simulink model "AUV_Multi_MPC"  (R2023a)
settings: Solver=ode23t  StartTime=0.0  StopTime=300  MaxStep=0.01  RelTol=1e-3  EnableMultiTasking=on
PreLoadFcn:
  | AUV_VehicleParameters;
  | Vehicle.Body.markeropacity = 0;
InitFcn:
  | %% ========================= SAMPLE TIME =========================
  | Ts = 0.1;
  | %% ========================= MPC: SURGE X =========================
  | nx = 1; nu = 1; ny = 1;
  | 
  | A = 0.9; B = 0.1; C = 1; D = 0;
  | plant = ss(A, B, C, D, Ts);
  | mpc1 = mpc(plant, Ts);
  | 
  | % Cấu hình như bình thường
  | mpc1.PredictionHorizon = 10;
  | mpc1.ControlHorizon = 2;
  | 
  | mpc1.Weights.OV = 7.5; % đủ mạnh để bám
  | mpc1.Weights.MV = 0.08; % cho dùng lực nhiều hơn
  | mpc1.Weights.MVRate = 0.25; % vừa mượt vừa linh hoạt
  | mpc1.MV.Min = -40;
  | mpc1.MV.Max = 40;
  | mpc1.OV.Min = 0;
  | mpc1.OV.Max = 2;
  | 
  | % Ràng buộc về thay đổi lực
  | mpc1.MV.RateMin = -12.5;
  | mpc1.MV.RateMax = 12.5;
  | %% ========================= MPC OUTER LOOP FOR DEPTH (Z) =========================
  | % ===== Baseline outer MPC for depth =====
  | u0 = 1.2;
  | 
  | A = 1;
  | B = -Ts*u0;
  | C = 1;
  | D = 0;
  | 
  | plant_z = ss(A,B,C,D,Ts);
  | 
  | mpc_z = mpc(plant_z,Ts);
  | mpc_z.PredictionHorizon = 10;
  | mpc_z.ControlHorizon    = 2;
  | 
  | mpc_z.Weights.OV     = 12;
  | mpc_z.Weights.MV     = 0.01;
  | mpc_z.Weights.MVRate = 0.1;
  | 
  | theta_ref_max = deg2rad(18);
  | mpc_z.MV.Min = -theta_ref_max;
  | mpc_z.MV.Max =  theta_ref_max;
  | 
  | mpc_z.MV.RateMin = -deg2rad(4);
  | mpc_z.MV.RateMax =  deg2rad(4);
  | 
  | 
  | %% ========================= MPC OUTER LOOP FOR HEADING =========================
  | A = 1;
  | B = Ts;
  | C = 1;
  | D = 0;
  | 
  | plant_psi = ss(A,B,C,D,Ts);
  | mpc_psi = mpc(plant_psi,Ts);
  | 
  | mpc_psi.PredictionHorizon = 10;
  | mpc_psi.ControlHorizon    = 2;
  | 
  | mpc_psi.Weights.OV     = 10;
  | mpc_psi.Weights.MV     = 0.05;
  | mpc_psi.Weights.MVRate = 1;
  | 
  | psidot_ref_max = deg2rad(20);
  | mpc_psi.MV.Min = -psidot_ref_max;
  | mpc_psi.MV.Max =  psidot_ref_max;
  | 
  | mpc_psi.MV.RateMin = -deg2rad(10);
  | mpc_psi.MV.RateMax =  deg2rad(10);
StopFcn:
  | try
  |     S = out;
  | 
  |     % ===============================
  |     % CHỌN HỆ QUY CHIẾU
  |     % ===============================
  |     USE_UP = true;   % true = ENU (Up), false = NED (Down)
  | 
  |     % ===============================
  |     % AUV position (NED gốc)
  |     % ===============================
  |     P  = squeeze(S.auv_position.signals.values);   % [Xn Ye Zd]
  |     tP = S.auv_position.time(:);
  | 
  |     Xn = P(:,1);   % North
  |     Ye = P(:,2);   % East
  |     Zd = P(:,3);   % Down (+)
  | 
  |     % ===============================
  |     % Reference vector
  |     % ===============================
  |     R = squeeze(S.auv_reference.signals.values);  % [V D psi]
  |     t = S.auv_reference.time(:);
  | 
  |     V   = R(:,1);      % speed
  |     D   = R(:,2);      % depth (Down +)
  |     psi = R(:,3);      % heading (rad)
  | 
  |     % ===============================
  |     % Reconstruct reference trajectory (NED)
  |     % ===============================
  |     Xr = Xn(1) + cumtrapz(t, V .* cos(psi));   % North
  |     Yr = Ye(1) + cumtrapz(t, V .* sin(psi));   % East
  |     Zr_down = Zd(1) + (D - D(1));              % Down (+)
  | 
  |     % ===============================
  |     % CHUYỂN HỆ (nếu cần)
  |     % ===============================
  |     if USE_UP
  |         Za  = -Zd;        % Up
  |         Zr  = -Zr_down;   % Up
  |         zlbl = 'Z (Up, m)';
  |     else
  |         Za  = Zd;         % Down
  |         Zr  = Zr_down;
  |         zlbl = 'Z (Down, m)';
  |     end
  | 
  |     % ===============================
  |     % Plot
  |     % ===============================
  |     f = figure(2); clf(f);
  |     set(f,'Name','AUV vs Reference','NumberTitle','off');
  | 
  |     ax = gca;
  |     ax.SortMethod = 'childorder';
  | 
  |     hRef   = plot3(Xr, Yr, Zr, '--', ...
  |                    'Color',[0.6 0.6 0.6], 'LineWidth',1.2);
  |     hold on
  | 
  |     hAUV   = plot3(Xn, Ye, Za, ...
  |                    'LineWidth',1.8, 'Color',[0 0.447 0.741]);
  | 
  |     hStart = plot3(Xn(1), Ye(1), Za(1),  'r*');
  |     hEnd   = plot3(Xn(end),Ye(end),Za(end),'g*');
  | 
  |     grid on;
  |     axis equal;
  |     view(45,25);
  | 
  |     xlabel('X (North, m)');
  |     ylabel('Y (East, m)');
  |     zlabel(zlbl);
  | 
  |     legend([hAUV hRef hStart hEnd], ...
  |            {'AUV','Reference','Start','End'}, ...
  |            'Location','best');
  | 
  |     drawnow;
  | 
  | catch ME
  |     warning('Plot AUV/Ref failed: %s', ME.message);
  | end
model workspace: external: MATLAB File AUV_DataFile_ORIG.m (data not in the file)
undefined symbols (not defined in the file): Environment, Newton, Raphson, smiData, x, X, Y, y, Z
libraries: sm_lib x3123, nesl_utility x51, sharedutil x8, simulink x6, AUVCustomPrimitives_Lib x4, mpclib x3, fuzblock x2, instrumentseriallib x2, shared6dof x1, slpidlib x1, aerolibasang x1, aerolibadyn x1
(part 1 of 72)
settings Model: Creator=cosorio  LastModifiedBy=antru
settings DataIOCC: MaxDataPoints=10000  SaveOutput=off  DSMLogging=off  SaveTime=off  SignalLoggingName=logsout_controls
settings OptimizationCC: LifeSpan=inf
settings DebuggingCC: UnconnectedInputMsg=warning  UnconnectedOutputMsg=warning  UnconnectedLineMsg=warning  AllowSymbolicDim=off  SFUnexpectedBacktrackingDiag=warning  SFNoUnconditionalDefaultTransitionDiag=warning  SFExecutionAtInitializationDiag=none  ArithmeticOperatorsInVariantConditions=warning
settings ModelReferenceCC: EnableRefExpFcnMdlSchedulingChecks=on
settings SFSimCC: SimUseLocalCustomCode=off  CustomCodeUndefinedFunction=UseInterfaceOnly
settings RTWCC: RTWUseLocalCustomCode=off  DLArmComputeVersion=19.05
settings CodeAppCC: StateflowObjectComments=on
settings GRTTargetCC: TargetLangStandard=C89/C90 (ANSI)
settings ConfigComp: CovMetricSettings=dw  CovSaveCumulativeToWorkspaceVar=on  CovSaveSingleToWorkspaceVar=on  CovExternalEMLEnable=off  CovSFcnEnable=off
settings SimscapeCC: SimscapeLogName=simlog_hydrodynamicsVAR  SimscapeLogLimitData=off  SimscapeLogDataHistory=10000
settings DiagnosticsConfigSet: SimMechanicsUnconnectedFramePorts=none  SimMechanicsConflictingReferenceFrames=none
settings ExplorerConfigSet: InternalSimMechanicsExplorerSettings="<ExplorerConfiguration><canonicalview>aerospace</canonicalview><AnimationSetting><BasePlaybackSpeed>1.0</BasePlaybackSpeed><PlaybackSpeedFactor>4.0</PlaybackSpeedFactor></AnimationSetting><TilePanel><TileInfo><Tiles Columns=\"2\" Count=\"4\" Rows=\"2\"><Column Weight=\"0.4992\"/><Column Weight=\"0.5008\"/><Row Weight=\"0.5\"/><Row Weight=\"0.5\"/><Tile Height=\"1\" Width=\"1\" X=\"0\" Y=\"0\"/><Tile Height=\"1\" Width=\"1\" X=\"0\" Y=\"1\"/><Tile Height=\"1\" Width=\"1\" X=\"1\" Y=\"0\"/><Tile Height=\"1\" Width=\"1\" X=\"1\" Y=\"1\"/></Tiles></TileInfo><SceneInfo><SceneViewer><BGColor><R>1</R><G>1</G><B>1</B></BGColor><Camera><DoPerspective>on</DoPerspective><Position><X>-3.00000146164778636</X><Y>7.03310812635629781e-05</Y><Z>2</Z></Position><Center><X>-1.46164778620002517e-06</X><Y>7.03310812637207838e-05</Y><Z>5</Z></Center><Up><X>0</X><Y>0</Y><Z>-1</Z></Up><ViewLimDist>1</ViewLimDist><YLim>0.466307658154998583</YLim><XLim>0.489133907155592906</XLim></Camera></SceneViewer><SceneViewer><BGColor><R>1</R><G>1</G><B>1</B></BGColor><Camera><DoPerspective>on</DoPerspective><Position><X>-1.46164778620001966e-06</X><Y>7.03310812635620566e-05</Y><Z>2</Z></Position><Center><X>-1.46164778620002517e-06</X><Y>7.03310812637207838e-05</Y><Z>5</Z></Center><Up><X>1</X><Y>0</Y><Z>0</Z></Up><ViewLimDist>1</ViewLimDist><YLim>0.466307658154998583</YLim><XLim>0.489133907155592906</XLim></Camera></SceneViewer><SceneViewer><BGColor><R>1</R><G>1</G><B>1</B></BGColor><Camera><DoPerspective>on</DoPerspective><Position><X>-2.50000146164778636</X><Y>-1.49992966891873625</Y><Z>2.5</Z></Position><Center><X>-1.46164778620002517e-06</X><Y>7.03310812637207838e-05</Y><Z>5</Z></Center><Up><X>0</X><Y>0</Y><Z>-1</Z></Up><ViewLimDist>1</ViewLimDist><YLim>0.466307658154998583</YLim><XLim>0.489133907155592906</XLim></Camera></SceneViewer><SceneViewer><BGColor><R>1</R><G>1</G><B>1</B></BGColor><Camera><DoPerspective>on</DoPerspective><Position><X>-1.46164778620094505e-06</X><Y>-2.99992966891873625</Y><Z>5</Z></Position><Center><X>-1.46164778620002517e-06</X><Y>7.03310812637207838e-05</Y><Z>5</Z></Center><Up><X>0</X><Y>0</Y><Z>-1</Z></Up><ViewLimDist>1</ViewLimDist><YLim>0.466307658154998583</YLim><XLim>0.489133907155592906</XLim></Camera></SceneViewer></SceneInfo></TilePanel><MechEditorPanel><Cameras><Camera><Id>Camera1</Id><Value><Name>Behind</Name><NativeCamera><PositionTrackingFeature>AUV.Muiltibody.Cameras.Behind.R</PositionTrackingFeature><CenterTrackingFeature>AUV.Muiltibody.Cameras.CoM</CenterTrackingFeature><UpVectorTrackingFeature>AUV.Muiltibody.World.W</UpVectorTrackingFeature><CenterTrackingOrigin>on</CenterTrackingOrigin><UpVectorTrackingDirection>-Z</UpVectorTrackingDirection></NativeCamera></Value></Camera><Camera><Id>Camera2</Id><Value><Name>BehindUP</Name><NativeCamera><PositionTrackingFeature>AUV.Muiltibody.Cameras.BehindUP.R</PositionTrackingFeature><CenterTrackingFeature>AUV.Muiltibody.Cameras.CoM</CenterTrackingFeature><UpVectorTrackingFeature>AUV.Muiltibody.World.W</UpVectorTrackingFeature><CenterTrackingOrigin>on</CenterTrackingOrigin><UpVectorTrackingDirection>-Z</UpVectorTrackingDirection></NativeCamera></Value></Camera><Camera><Id>Camera3</Id><Value><Name>BehindDown</Name><NativeCamera><PositionTrackingFeature>AUV.Muiltibody.Cameras.BehindDown.R</PositionTrackingFeature><CenterTrackingFeature>AUV.Muiltibody.Cameras.CoM</CenterTrackingFeature><UpVectorTrackingFeature>AUV.Muiltibody.World.W</UpVectorTrackingFeature><CenterTrackingOrigin>on</CenterTrackingOrigin><UpVectorTrackingDirection>-Z</UpVectorTrackingDirection></NativeCamera></Value></Camera><Camera><Id>Camera4</Id><Value><Name>BehindUPLeft</Name><NativeCamera><PositionTrackingFeature>AUV.Muiltibody.Cameras.BehindUPLeft.R</PositionTrackingFeature><CenterTrackingFeature>AUV.Muiltibody.Cameras.CoM</CenterTrackingFeature><UpVectorTrackingFeature>AUV.Muiltibody.World.W</UpVectorTrackingFeature><CenterTrackingOrigin>on</CenterTrackingOrigin><UpVectorTrackingDirection>-Z</UpVectorTrackingDirection></NativeCamera></Value></Camera><Camera><Id>Camera5</Id><Value><Name>BehindUPRight</Name><NativeCamera><PositionTrackingFeature>AUV.Muiltibody.Cameras.BehindUPRight.R</PositionTrackingFeature><CenterTrackingFeature>AUV.Muiltibody.Cameras.CoM</CenterTrackingFeature><UpVectorTrackingFeature>AUV.Muiltibody.World.W</UpVectorTrackingFeature><CenterTrackingOrigin>on</CenterTrackingOrigin><UpVectorTrackingDirection>-Z</UpVectorTrackingDirection></NativeCamera></Value></Camera><Camera><Id>Camera6</Id><Value><Name>Top</Name><NativeCamera><PositionTrackingFeature>AUV.Muiltibody.Cameras.Top.R</PositionTrackingFeature><CenterTrackingFeature>AUV.Muiltibody.Cameras.CoM</CenterTrackingFeature><UpVectorTrackingFeature>AUV.Muiltibody.World.W</UpVectorTrackingFeature><CenterTrackingOrigin>on</CenterTrackingOrigin><UpVectorTrackingDirection>+X</UpVectorTrackingDirection></NativeCamera></Value></Camera><Camera><Id>Camera7</Id><Value><Name>Side</Name><NativeCamera><PositionTrackingFeature>AUV.Muiltibody.Cameras.Side.R</PositionTrackingFeature><CenterTrackingFeature>AUV.Muiltibody.Cameras.CoM</CenterTrackingFeature><UpVectorTrackingFeature>AUV.Muiltibody.World.W</UpVectorTrackingFeature><CenterTrackingOrigin>on</CenterTrackingOrigin><UpVectorTrackingDirection>-Z</UpVectorTrackingDirection></NativeCamera></Value></Camera><Camera><Id>Camera8</Id><Value><Name>ISO</Name><NativeCamera><PositionTrackingFeature>AUV.Muiltibody.Cameras.ISO.R</PositionTrackingFeature><CenterTrackingFeature>AUV.Muiltibody.Cameras.CoM</CenterTrackingFeature><UpVectorTrackingFeature>AUV.Muiltibody.Cameras.World.W</UpVectorTrackingFeature><CenterTrackingOrigin>on</CenterTrackingOrigin><UpVectorTrackingDirection>-Z</UpVectorTrackingDirection></NativeCamera></Value></Camera></Cameras><GfxPanelCameraMap><MapElement CameraMLId=\"Camera2\" GfxPanelIndex=\"0\"/><MapElement CameraMLId=\"Camera6\" GfxPanelIndex=\"1\"/><MapElement CameraMLId=\"Camera8\" GfxPanelIndex=\"2\"/><MapElement CameraMLId=\"Camera7\" GfxPanelIndex=\"3\"/></GfxPanelCameraMap><VideoCreator><PlaybackSpeedRatio>1.0</PlaybackSpeedRatio><FrameRate>30</FrameRate><VideoFormat>Motion JPEG AVI</VideoFormat><FrameSize>auto</FrameSize></VideoCreator></MechEditorPanel></ExplorerConfiguration>"

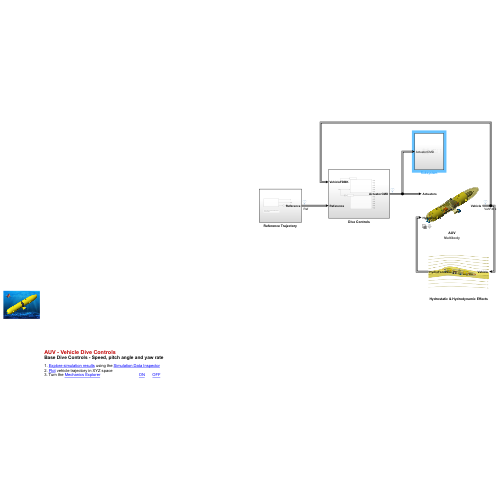
[thumbnail: Simulink's stored preview of the top-level diagram]
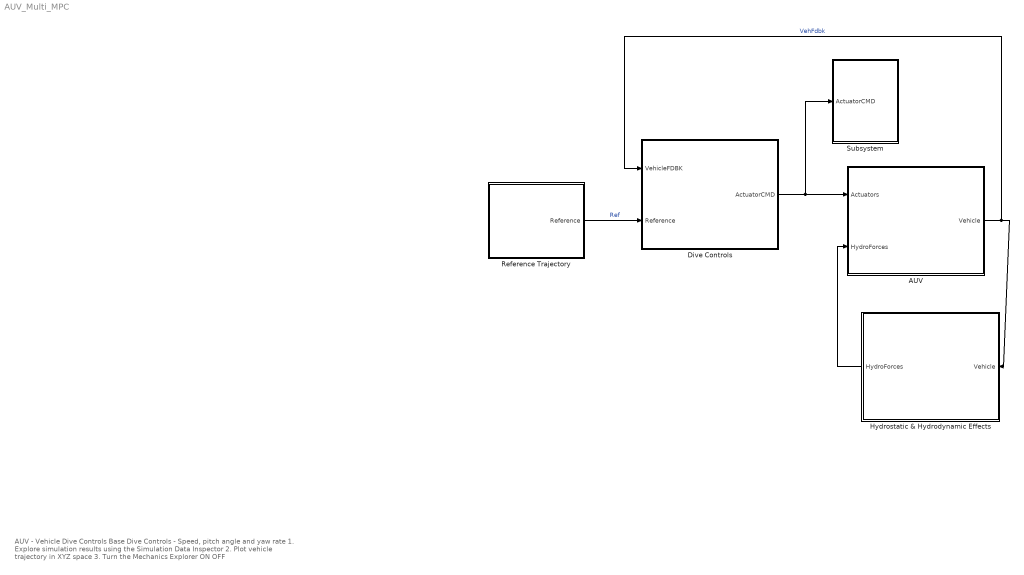
== system AUV_Multi_MPC ==
  note: AUV - Vehicle Dive Controls
      | Base Dive Controls - Speed, pitch angle and yaw rate
      |
      | 1. Explore simulation results using the Simulation Data Inspector
      | 2. Plot vehicle trajectory in XYZ space
      | 3. Turn the Mechanics Explorer ON OFF
  AUV : Subsystem  Variant=on  VariantControlMode=label  VariantControl=Choice  LabelModeActiveChoice=Multibody  mask(AUV){VariantLabel=Multibody}
      mask prompts: VariantLabel "Select Variant:"
      mask help:
      | These block contains two variant implementations of the equations of motion for the rigid body dynamics of the underwater vehicle:
      | Multibody Variant  : implements the dynamics using CAD files and Simscape Multibody
      | Singlebody Variant : implements the dynamics using the 6-DoF block from Aerospace Blockset
      mask init:
      | % Set active variant choice for this block
      | if VariantLabel == 1
      |     ActiveChoice = 'Multibody';
      | else
      |     ActiveChoice = 'Singlebody';
      | end
      | 
      | set_param(gcb,'LabelModeActiveChoice',ActiveChoice);
      settings: AttributesFormatString=%<LabelModeActiveChoice>
      mask TypeOptions VariantLabel: Multibody | Singlebody
      mask Display:
      | blk = find_system(gcbh, 'LookUnderMasks', 'all', 'SearchDepth', 1,'FollowLinks','on', 'Parent', gcb,'VariantObject', get_param(gcb,'activevariant'));
      | eval(get_param(blk, 'MaskDisplay'));
  Dive Controls : Subsystem
  Hydrostatic & Hydrodynamic Effects : Subsystem
      mask Display: image('Drag.png',[0,0.15,1,0.7])
  Reference Trajectory : Subsystem
  Subsystem : Subsystem
  wires:
  Reference Trajectory/1(Reference) -> Dive Controls/2(Reference)  "Ref"
  Hydrostatic & Hydrodynamic Effects/1(HydroForces) -> AUV/2(HydroForces)
  AUV/1(Vehicle) -> Dive Controls/1(VehicleFDBK), Hydrostatic & Hydrodynamic Effects/1(Vehicle)  "VehFdbk"
  Dive Controls/1(ActuatorCMD) -> Subsystem/1(ActuatorCMD), AUV/1(Actuators)

== system AUV_Multi_MPC/AUV ==
  Actuators : Inport
  HydroForces : Inport  Port=2
  Muiltibody : Subsystem  VariantControl=Multibody
      mask Display: image('AUV.png',[0.05,0,0.9,1])
  Singlebody : Subsystem  VariantControl=Singlebody
      mask Display: image('AUVEllipsoid.png',[0.05,0,0.9,1])
  Vehicle : Outport

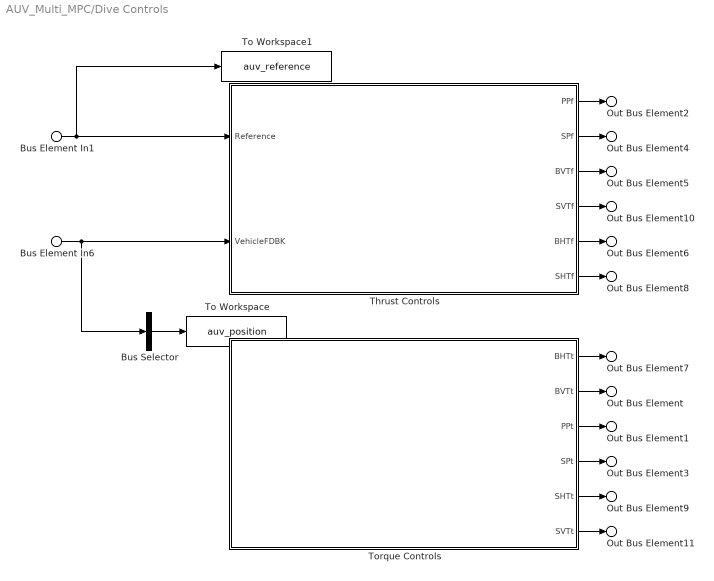
== system AUV_Multi_MPC/Dive Controls ==
  Bus Element In6 : Inport  PortName=VehicleFDBK
  Bus Element In1 : Inport  Port=2  PortName=Reference
  Bus Selector : BusSelector  OutputSignals=CoM.World.Xe  OutputAsBus=on
  Thrust Controls : Subsystem
  To Workspace : ToWorkspace  VariableName=auv_position  SaveFormat=Structure With Time  SampleTime=-1
  To Workspace1 : ToWorkspace  VariableName=auv_reference  SaveFormat=Structure With Time  SampleTime=-1
  Torque Controls : Subsystem
  Out Bus Element2 : Outport  PortName=ActuatorCMD  Element=Propellers.PPf
  Out Bus Element1 : Outport  PortName=ActuatorCMD  Element=Propellers.PPt
  Out Bus Element4 : Outport  PortName=ActuatorCMD  Element=Propellers.SPf
  Out Bus Element3 : Outport  PortName=ActuatorCMD  Element=Propellers.SPt
  Out Bus Element6 : Outport  PortName=ActuatorCMD  Element=Thrusters.BHTf
  Out Bus Element7 : Outport  PortName=ActuatorCMD  Element=Thrusters.BHTt
  Out Bus Element5 : Outport  PortName=ActuatorCMD  Element=Thrusters.BVTf
  Out Bus Element : Outport  PortName=ActuatorCMD  Element=Thrusters.BVTt
  Out Bus Element8 : Outport  PortName=ActuatorCMD  Element=Thrusters.SHTf
  Out Bus Element9 : Outport  PortName=ActuatorCMD  Element=Thrusters.SHTt
  Out Bus Element10 : Outport  PortName=ActuatorCMD  Element=Thrusters.SVTf
  Out Bus Element11 : Outport  PortName=ActuatorCMD  Element=Thrusters.SVTt
  wires:
  Torque Controls/1(BHTt) -> Out Bus Element7/1
  Torque Controls/2(BVTt) -> Out Bus Element/1
  Torque Controls/3(PPt) -> Out Bus Element1/1
  Torque Controls/4(SPt) -> Out Bus Element3/1
  Torque Controls/5(SHTt) -> Out Bus Element9/1
  Torque Controls/6(SVTt) -> Out Bus Element11/1
  Thrust Controls/3(BVTf) -> Out Bus Element5/1
  Thrust Controls/4(SVTf) -> Out Bus Element10/1
  Thrust Controls/5(BHTf) -> Out Bus Element6/1
  Thrust Controls/6(SHTf) -> Out Bus Element8/1
  Thrust Controls/1(PPf) -> Out Bus Element2/1
  Thrust Controls/2(SPf) -> Out Bus Element4/1
  Bus Element In1/1 -> To Workspace1/1, Thrust Controls/1(Reference)
  Bus Element In6/1 -> Bus Selector/1, Thrust Controls/2(VehicleFDBK)
  Bus Selector/1 -> To Workspace/1

== system AUV_Multi_MPC/Hydrostatic & Hydrodynamic Effects ==
  Bus Element In1 : Inport  PortName=Vehicle  Element=CoM.Body.Vb
  Bus Element In2 : Inport  PortName=Vehicle  Element=CoM.Body.wb
  Bus Element In3 : Inport  PortName=Vehicle  Element=CoM.Body.dwbdt
  Bus Element In4 : Inport  PortName=Vehicle  Element=CoM.Derived.Body.Abb
  Bus Element In5 : Inport  PortName=Vehicle  Element=CoM.Derived.Body.Incidences
  Added Mass Forces : Subsystem
  Buoyancy (N) : Constant  Value=Vehicle.Body.Full.buoyancyforce
  Hydrostatic Forces : Subsystem
  Lift and Drag Forces : Subsystem
  Sea Water Density (kg/m^3) : Constant  Value=Environment.seawaterdensity
  Underwater Current Forces : Subsystem
  Weight (N) : Constant  Value=Vehicle.Body.Full.totalweight
  Bus Element Out : Outport  PortName=HydroForces  Element=Buoyancy
  Bus Element Out1 : Outport  PortName=HydroForces  Element=LiftNDrag
  Bus Element Out2 : Outport  PortName=HydroForces  Element=AddedMass
  Bus Element Out3 : Outport  PortName=HydroForces  Element=UnderwaterCurrent
  Bus Element Out4 : Outport  PortName=HydroForces  Element=Weight
  wires:
  Sea Water Density (kg/m^3)/1 -> Lift and Drag Forces/1(rho)
  Bus Element In1/1 -> Lift and Drag Forces/3(Vb), Added Mass Forces/1(Vb)
  Buoyancy (N)/1 -> Hydrostatic Forces/1(B)
  Bus Element In2/1 -> Lift and Drag Forces/4(wb), Added Mass Forces/2(wb)
  Bus Element In4/1 -> Added Mass Forces/3(Abb)
  Bus Element In3/1 -> Added Mass Forces/4(dwbdt)
  Bus Element In5/1 -> Lift and Drag Forces/2(alpha,beta)
  Hydrostatic Forces/1(Buoyancy) -> Bus Element Out/1
  Lift and Drag Forces/1(LiftNDrag) -> Bus Element Out1/1
  Added Mass Forces/1(AddedMass) -> Bus Element Out2/1
  Underwater Current Forces/1(UnderwaterCurrent) -> Bus Element Out3/1
  Weight (N)/1 -> Hydrostatic Forces/2(W)
  Hydrostatic Forces/2(Weight) -> Bus Element Out4/1

== system AUV_Multi_MPC/Reference Trajectory ==
  note: NOTE: Double-click on the Reference Trajectory block to choose the different Active Scenario available.
  Reference Trajectory : SignalEditorBlockLib/Signal Editor  FileName=RefTrajectory.mat  ActiveScenario=StraightDiveNTurn  ActiveSignal=Speed  IsBus=off  OutputBusObjectStr=Bus: BusObject  SampleTime=0  OutputAfterFinalValue=Holding final value  Unit=inherit  PreserveSignalName=on  ApplySigPropsToAllScenarios=on
  deg2rad : Gain  Gain=pi/180
  Out Bus Element2 : Outport  PortName=Reference  Element=Speed
  Out Bus Element1 : Outport  PortName=Reference  Element=Depth
  Out Bus Element3 : Outport  PortName=Reference  Element=Heading
  wires:
  Reference Trajectory/1 -> Out Bus Element2/1
  Reference Trajectory/2 -> Out Bus Element1/1
  Reference Trajectory/3 -> deg2rad/1
  deg2rad/1 -> Out Bus Element3/1

== system AUV_Multi_MPC/Subsystem ==
  In Bus Element : Inport  PortName=ActuatorCMD  Element=Propellers.PPf
  In Bus Element1 : Inport  PortName=ActuatorCMD  Element=Propellers.SPf
  In Bus Element2 : Inport  PortName=ActuatorCMD  Element=Thrusters.BHTf
  In Bus Element3 : Inport  PortName=ActuatorCMD  Element=Thrusters.BVTf
  In Bus Element4 : Inport  PortName=ActuatorCMD  Element=Thrusters.SVTf
  In Bus Element5 : Inport  PortName=ActuatorCMD  Element=Thrusters.SHTf
  Compare To Constant{,1..5} (6 alike) : simulink/Logic and Bit Operations/Compare To Constant  relop=>=  const=1  OutDataTypeStr=uint8
  Display1 : Display
  MATLAB Function : MATLAB Function  TreatAsAtomicUnit=on
  Serial Configuration : instrumentseriallib/Serial Configuration  Priority=-200000  PortSel=COM6  Port=COM6  ComPort=COM6  BaudRate=9600  DataBits=8  Parity=none  StopBits=1  ByteOrder=little-endian  FlowControl=none  Timeout=10  SimulateUsing=Interpreted execution  BlockInModel=on  aMode=1
  Serial Send : instrumentseriallib/Serial Send  Priority=1  PortSel=COM6  Port=COM6  ComPort=COM6  Header=[]  Terminator=<none>  CustomTerminator=[]  EnableBlockingMode=on  SimulateUsing=Interpreted execution  BlockInModel=on  aMode=1
  wires:
  In Bus Element/1 -> Compare To Constant/1
  In Bus Element1/1 -> Compare To Constant1/1
  In Bus Element3/1 -> Compare To Constant2/1
  In Bus Element4/1 -> Compare To Constant3/1
  In Bus Element2/1 -> Compare To Constant4/1
  In Bus Element5/1 -> Compare To Constant5/1
  Compare To Constant/1 -> MATLAB Function/1(a)
  Compare To Constant1/1 -> MATLAB Function/2(b)
  Compare To Constant2/1 -> MATLAB Function/3(c)
  Compare To Constant3/1 -> MATLAB Function/4(d)
  Compare To Constant4/1 -> MATLAB Function/5(e)
  Compare To Constant5/1 -> MATLAB Function/6(f)
  MATLAB Function/1(cmd) -> Serial Send/1, Display1/1

== system AUV_Multi_MPC/AUV/Muiltibody ==
  Actuators : Inport
  HydroForces : Inport  Port=2
  6-DOF : sm_lib/Joints/6-DOF Joint  JointMode=Normal  SenseConstraintForce=off  SenseConstraintForceX=off  SenseConstraintForceY=off  SenseConstraintForceZ=off  SenseConstraintTorque=off  SenseConstraintTorqueX=off  SenseConstraintTorqueY=off  SenseConstraintTorqueZ=off  SenseTotalForce=off  SenseTotalForceX=off  SenseTotalForceY=off  SenseTotalForceZ=off  SenseTotalTorque=off  SenseTotalTorqueX=off  SenseTotalTorqueY=off  SenseTotalTorqueZ=off  CompositeWrenchDir=FollowerOnBase  CompositeWrenchFrame=FollowerFrame  PxEquilibriumPosition=0  PxEquilibriumPositionUnits=m  PxSpringStiffness=0  PxSpringStiffnessUnits=N/m  PxDampingCoefficient=0  PxDampingCoefficientUnits=N/(m/s)  PxTorqueActuationMode=NoTorque  PxMotionActuationMode=ComputedMotion  PxSensePosition=off  PxSenseVelocity=off  PxSenseAcceleration=off  PxSenseTorqueForce=off  PxSenseLowerLimitTorqueForce=off  PxSenseUpperLimitTorqueForce=off  PxLowerLimitSpecify=off  PxLowerLimitBound=-1  PxLowerLimitBoundUnits=m  PxLowerLimitStiffness=1e6  PxLowerLimitStiffnessUnits=N/m  PxLowerLimitDamping=1e3  PxLowerLimitDampingUnits=N/(m/s)  PxLowerLimitTransitionRegionWidth=1e-4  PxLowerLimitTransitionRegionWidthUnits=m  PxUpperLimitSpecify=off  PxUpperLimitBound=1  PxUpperLimitBoundUnits=m  PxUpperLimitStiffness=1e6  PxUpperLimitStiffnessUnits=N/m  PxUpperLimitDamping=1e3  PxUpperLimitDampingUnits=N/(m/s)  PxUpperLimitTransitionRegionWidth=1e-4  PxUpperLimitTransitionRegionWidthUnits=m  PxPositionTargetSpecify=off  PxPositionTargetPriority=High  PxPositionTargetValue=0  PxPositionTargetValueUnits=m  PxVelocityTargetSpecify=off  PxVelocityTargetPriority=High  PxVelocityTargetValue=0  PxVelocityTargetValueUnits=m/s  PyEquilibriumPosition=0  PyEquilibriumPositionUnits=m  PySpringStiffness=0  PySpringStiffnessUnits=N/m  PyDampingCoefficient=0  PyDampingCoefficientUnits=N/(m/s)  PyTorqueActuationMode=NoTorque  PyMotionActuationMode=ComputedMotion  PySensePosition=off  PySenseVelocity=off  PySenseAcceleration=off  PySenseTorqueForce=off  PySenseLowerLimitTorqueForce=off  PySenseUpperLimitTorqueForce=off  PyLowerLimitSpecify=off  PyLowerLimitBound=-1  PyLowerLimitBoundUnits=m  PyLowerLimitStiffness=1e6  PyLowerLimitStiffnessUnits=N/m  PyLowerLimitDamping=1e3  PyLowerLimitDampingUnits=N/(m/s)  PyLowerLimitTransitionRegionWidth=1e-4  PyLowerLimitTransitionRegionWidthUnits=m  PyUpperLimitSpecify=off  PyUpperLimitBound=1  PyUpperLimitBoundUnits=m  PyUpperLimitStiffness=1e6  PyUpperLimitStiffnessUnits=N/m  PyUpperLimitDamping=1e3  PyUpperLimitDampingUnits=N/(m/s)  PyUpperLimitTransitionRegionWidth=1e-4  PyUpperLimitTransitionRegionWidthUnits=m  PyPositionTargetSpecify=off  PyPositionTargetPriority=High  PyPositionTargetValue=0  PyPositionTargetValueUnits=m  PyVelocityTargetSpecify=off  PyVelocityTargetPriority=High  PyVelocityTargetValue=0  PyVelocityTargetValueUnits=m/s  PzEquilibriumPosition=0  PzEquilibriumPositionUnits=m  PzSpringStiffness=0  PzSpringStiffnessUnits=N/m  PzDampingCoefficient=0  PzDampingCoefficientUnits=N/(m/s)  PzTorqueActuationMode=NoTorque  PzMotionActuationMode=ComputedMotion  PzSensePosition=off  PzSenseVelocity=off  PzSenseAcceleration=off  PzSenseTorqueForce=off  PzSenseLowerLimitTorqueForce=off  PzSenseUpperLimitTorqueForce=off  PzLowerLimitSpecify=off  PzLowerLimitBound=-1  PzLowerLimitBoundUnits=m  PzLowerLimitStiffness=1e6  PzLowerLimitStiffnessUnits=N/m  PzLowerLimitDamping=1e3  PzLowerLimitDampingUnits=N/(m/s)  PzLowerLimitTransitionRegionWidth=1e-4  PzLowerLimitTransitionRegionWidthUnits=m  PzUpperLimitSpecify=off  PzUpperLimitBound=1  PzUpperLimitBoundUnits=m  PzUpperLimitStiffness=1e6  PzUpperLimitStiffnessUnits=N/m  PzUpperLimitDamping=1e3  PzUpperLimitDampingUnits=N/(m/s)  PzUpperLimitTransitionRegionWidth=1e-4  PzUpperLimitTransitionRegionWidthUnits=m  PzPositionTargetSpecify=on  PzPositionTargetPriority=High  PzPositionTargetValue=Vehicle.InitCond.position(3)  PzPositionTargetValueUnits=m  PzVelocityTargetSpecify=off  PzVelocityTargetPriority=High  PzVelocityTargetValue=0  PzVelocityTargetValueUnits=m/s  SphEqPosRotationMethod=None  SphEqPosRotationAngleUnits=deg  SphEqPosRotationStandardAxis=+Z  SphEqPosRotationAngle=0.0  SphEqPosRotationArbitraryAxis=[0 0 1]  SphEqPosFollAlignAxisA=+X  SphEqPosBaseAlignAxisA=+Y  SphEqPosFollAlignAxisB=+Y  SphEqPosBaseAlignAxisB=+Z  SphEqPosRotationSequenceAxes=FollowerAxes  SphEqPosRotationSequence=XYX  SphEqPosRotationSequenceAngles=[0 0 0]  SphEqPosRotationSequenceAnglesUnits=deg  SphEqPosRotationMatrix=[1 0 0; 0 1 0; 0 0 1]  SphEqPosQuaternion=[1 0 0 0]  SphSpringStiffness=0  SphSpringStiffnessUnits=N*m/deg  SphDampingCoefficient=0  SphDampingCoefficientUnits=N*m/(deg/s)  SphActuateTorqueX=off  SphActuateTorqueY=off  SphActuateTorqueZ=off  SphActuateTorque=off  SphTorqueActuationMode=NoTorque  SphMotionActuationMode=ComputedMotion  SphActuationFrame=BaseFrame  SphSensePosition=off  SphSenseVelocityX=off  SphSenseVelocityY=off  SphSenseVelocityZ=off  SphSenseVelocity=off  SphSenseAccelerationX=off  SphSenseAccelerationY=off  SphSenseAccelerationZ=off  SphSenseAcceleration=off  SphSenseTorqueX=off  SphSenseTorqueY=off  SphSenseTorqueZ=off  SphSenseTorqueForce=off  SphSenseLowerLimitTorqueMag=off  SphSenseUpperLimitTorqueMag=off  SphSensingFrame=BaseFrame  SphLowerLimitSpecify=off  SphLowerLimitBound=15  SphLowerLimitBoundUnits=deg  SphLowerLimitStiffness=1e4  SphLowerLimitStiffnessUnits=N*m/deg  SphLowerLimitDamping=10  SphLowerLimitDampingUnits=N*m/(deg/s)  SphLowerLimitTransitionRegionWidth=0.1  SphLowerLimitTransitionRegionWidthUnits=deg  SphUpperLimitSpecify=off  SphUpperLimitBound=45  SphUpperLimitBoundUnits=deg  SphUpperLimitStiffness=1e4  SphUpperLimitStiffnessUnits=N*m/deg  SphUpperLimitDamping=10  SphUpperLimitDampingUnits=N*m/(deg/s)  SphUpperLimitTransitionRegionWidth=0.1  SphUpperLimitTransitionRegionWidthUnits=deg  SphPositionTargetRotationMethod=RotationMatrix  SphPositionTargetRotationAngleUnits=deg  SphPositionTargetRotationStandardAxis=+Z  SphPositionTargetRotationAngle=0.0  SphPositionTargetRotationArbitraryAxis=[0 0 1]  SphPositionTargetFollAlignAxisA=+X  SphPositionTargetBaseAlignAxisA=+Y  SphPositionTargetFollAlignAxisB=+Y  SphPositionTargetBaseAlignAxisB=+Z  SphPositionTargetRotationSequenceAxes=BaseAxes  SphPositionTargetRotationSequence=XYX  SphPositionTargetRotationSequenceAngles=[0 0 0]  SphPositionTargetRotationSequenceAnglesUnits=deg  SphPositionTargetRotationMatrix=Vehicle.InitCond.RotMZYX  SphPositionTargetQuaternion=[1 0 0 0]  SphPositionTargetSpecify=on  SphPositionTargetPriority=High  SphVelocityTargetValue=[0 0 0]  SphVelocityTargetValueUnits=deg/s  SphVelocityTargetSpecify=off  SphVelocityTargetPriority=High  SphVelocityTargetInFollowerFrame=on
  AUV Mechanics : Subsystem
      mask Display: image('AUVMechanics.png',[0.05,0.25,0.9,0.5])
  Cameras : Subsystem
  Hydro Forces & Moments : Subsystem
  World : Subsystem
  Vehicle : Outport
  wires:
  AUV Mechanics/1(Vehicle) -> Vehicle/1
  Actuators/1 -> AUV Mechanics/1(Actuators)
  HydroForces/1 -> Hydro Forces & Moments/1(HydroForces)
  connections:
  6-DOF/LConn1 -- World/RConn1
  6-DOF/RConn1 -- Hydro Forces & Moments/RConn1 -- Cameras/RConn1 -- AUV Mechanics/LConn1
  Hydro Forces & Moments/RConn2 -- AUV Mechanics/LConn2

== system AUV_Multi_MPC/AUV/Singlebody ==
  Actuators : Inport
  HydroForces : Inport  Port=2
  AUV Mechanics : Subsystem
  Hydro Forces & Moments : Subsystem
  Propellers & Thrusters : Subsystem
  Sum : Sum  Inputs=|++
  Sum1 : Sum  Inputs=++|
  Bus Element Out : Outport  PortName=Vehicle  Element=CoM
  wires:
  HydroForces/1 -> Hydro Forces & Moments/1(HydroForces)
  AUV Mechanics/1(CoM) -> Bus Element Out/1, Hydro Forces & Moments/2(CoM)
  Sum/1 -> AUV Mechanics/1(Fxyz)
  Hydro Forces & Moments/1(Fxyz) -> Sum/2
  Hydro Forces & Moments/2(Mxyz) -> Sum1/2
  Sum1/1 -> AUV Mechanics/2(Mxyz)
  Propellers & Thrusters/1(Fxyz) -> Sum/1
  Propellers & Thrusters/2(Mxyz) -> Sum1/1
  Actuators/1 -> Propellers & Thrusters/1(Actuators)

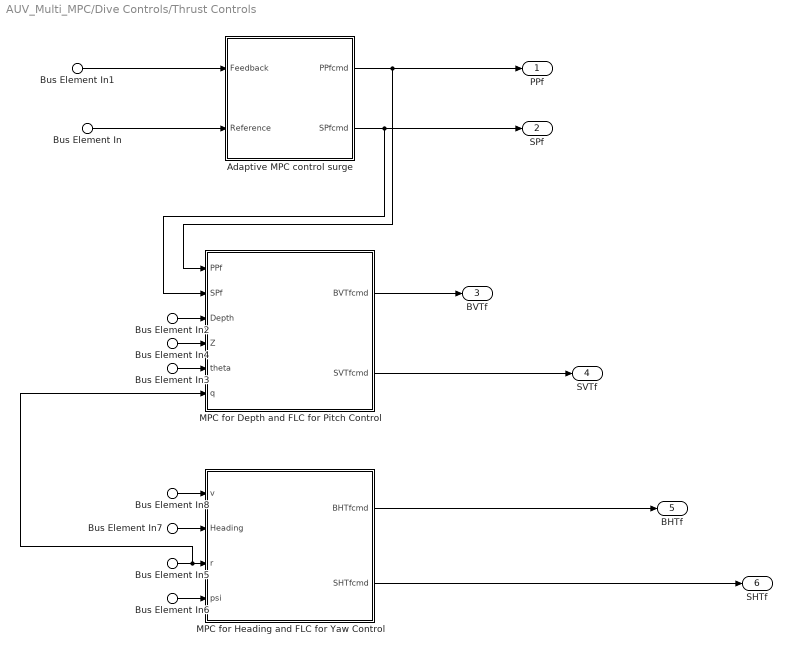
== system AUV_Multi_MPC/Dive Controls/Thrust Controls ==
  Bus Element In : Inport  PortName=Reference  Element=Speed
  Bus Element In2 : Inport  PortName=Reference  Element=Depth
  Bus Element In7 : Inport  PortName=Reference  Element=Heading
  Bus Element In1 : Inport  Port=2  PortName=VehicleFDBK  Element=CoM.Body.Vb.u
  Bus Element In8 : Inport  Port=2  PortName=VehicleFDBK  Element=CoM.Body.Vb.v
  Bus Element In5 : Inport  Port=2  PortName=VehicleFDBK  Element=CoM.Body.wb
  Bus Element In3 : Inport  Port=2  PortName=VehicleFDBK  Element=CoM.Derived.Euler.theta
  Bus Element In6 : Inport  Port=2  PortName=VehicleFDBK  Element=CoM.Derived.Euler.psi
  Bus Element In4 : Inport  Port=2  PortName=VehicleFDBK  Element=CoM.World.Xe.Z
  Adaptive MPC control surge : Subsystem
  MPC for Depth and FLC for Pitch Control : Subsystem
  MPC for Heading and FLC for Yaw Control : Subsystem
  PPf : Outport
  SPf : Outport  Port=2
  BVTf : Outport  Port=3
  SVTf : Outport  Port=4
  BHTf : Outport  Port=5
  SHTf : Outport  Port=6
  wires:
  MPC for Depth and FLC for Pitch Control/2(SVTfcmd) -> SVTf/1
  MPC for Depth and FLC for Pitch Control/1(BVTfcmd) -> BVTf/1
  MPC for Heading and FLC for Yaw Control/1(BHTfcmd) -> BHTf/1
  MPC for Heading and FLC for Yaw Control/2(SHTfcmd) -> SHTf/1
  Bus Element In2/1 -> MPC for Depth and FLC for Pitch Control/3(Depth)
  Bus Element In3/1 -> MPC for Depth and FLC for Pitch Control/5(theta)
  Bus Element In4/1 -> MPC for Depth and FLC for Pitch Control/4(Z)
  Bus Element In5/1 -> MPC for Heading and FLC for Yaw Control/3(r), MPC for Depth and FLC for Pitch Control/6(q)
  Bus Element In6/1 -> MPC for Heading and FLC for Yaw Control/4(psi)
  Bus Element In7/1 -> MPC for Heading and FLC for Yaw Control/2(Heading)
  Bus Element In8/1 -> MPC for Heading and FLC for Yaw Control/1(v)
  Adaptive MPC control surge/1(PPfcmd) -> MPC for Depth and FLC for Pitch Control/1(PPf), PPf/1
  Adaptive MPC control surge/2(SPfcmd) -> MPC for Depth and FLC for Pitch Control/2(SPf), SPf/1
  Bus Element In/1 -> Adaptive MPC control surge/2(Reference)
  Bus Element In1/1 -> Adaptive MPC control surge/1(Feedback)

== system AUV_Multi_MPC/Dive Controls/Torque Controls ==
  Tbht (N*m) : Constant  Value=0
  Tbvt (N*m) : Constant  Value=0
  Tpp (N*m) : Constant  Value=0
  Tsht (N*m) : Constant  Value=0
  Tsp (N*m) : Constant  Value=0
  Tsvt (N*m) : Constant  Value=0
  BHTt : Outport
  BVTt : Outport  Port=2
  PPt : Outport  Port=3
  SPt : Outport  Port=4
  SHTt : Outport  Port=5
  SVTt : Outport  Port=6
  wires:
  Tbht (N*m)/1 -> BHTt/1
  Tsvt (N*m)/1 -> SVTt/1
  Tpp (N*m)/1 -> PPt/1
  Tsp (N*m)/1 -> SPt/1
  Tbvt (N*m)/1 -> BVTt/1
  Tsht (N*m)/1 -> SHTt/1

== system AUV_Multi_MPC/Hydrostatic & Hydrodynamic Effects/Added Mass Forces ==
  Vb : Inport
  wb : Inport  Port=2
  Abb : Inport  Port=3
  dwbdt : Inport  Port=4
  Added Mass : Subsystem
  Added Mass Matrix : Constant  Value=Vehicle.AddedMass
  Coriolis : Subsystem
  Bus Element Out : Outport  PortName=AddedMass  Element=AMForcesXYZ
  Bus Element Out1 : Outport  PortName=AddedMass  Element=AMMomentsXYZ
  Bus Element Out2 : Outport  PortName=AddedMass  Element=CForcesXYZ
  Bus Element Out3 : Outport  PortName=AddedMass  Element=CMomentsXYZ
  wires:
  Added Mass Matrix/1 -> Added Mass/1(Ma), Coriolis/3(Ma)
  Abb/1 -> Added Mass/2(Abb)
  dwbdt/1 -> Added Mass/3(dwbdt)
  Added Mass/1(Fxyz) -> Bus Element Out/1
  Added Mass/2(Mxyz) -> Bus Element Out1/1
  Vb/1 -> Coriolis/1(Vb)
  wb/1 -> Coriolis/2(wb)
  Coriolis/2(Mxyz) -> Bus Element Out3/1
  Coriolis/1(Fxyz) -> Bus Element Out2/1

== system AUV_Multi_MPC/Hydrostatic & Hydrodynamic Effects/Hydrostatic Forces ==
  note: NOTE:
      | The vehicle is assumed to be fully submerged at all times
  B : Inport
  W : Inport  Port=2
  Bus Element Out : Outport  PortName=Buoyancy  Element=BForceZ
  Bus Element Out1 : Outport  Port=2  PortName=Weight  Element=WForceZ
  wires:
  B/1 -> Bus Element Out/1
  W/1 -> Bus Element Out1/1

== system AUV_Multi_MPC/Hydrostatic & Hydrodynamic Effects/Lift and Drag Forces ==
  note: NOTE:
      | We are assuming all hydrodynamic coefficients have been
      | computed with respect to the body center of mass, are
      | aligned with the body axes, and were normalized using the
      | front area of the vehicle as reference.
  rho : Inport
  alpha,beta : Inport  Port=2
  Vb : Inport  Port=3
  wb : Inport  Port=4
  CG : Constant  Value=[0,0,0]
  Dynamic Pressure : aerolibasang/Dynamic Pressure
  "Hydrodynamic Forces and Moments " : aerolibadyn/Aerodynamic Forces and Moments   inputAxes=Body  outputForceAxes=Body  outputMomentAxes=Body  S=Vehicle.Body.YZArea  b=Vehicle.Body.hulldiameter  cbar=Vehicle.Body.totallength
  Hydrodynamic Coefficients : Subsystem
  Scope : Scope
  Bus Element Out : Outport  PortName=LiftNDrag  Element=LDForcesXYZ
  Bus Element Out1 : Outport  PortName=LiftNDrag  Element=LDMomentsXYZ
  wires:
  rho/1 -> Dynamic Pressure/2
  Dynamic Pressure/1 -> "Hydrodynamic Forces and Moments "/2
  Vb/1 -> Dynamic Pressure/1, Hydrodynamic Coefficients/3(Vb)
  "Hydrodynamic Forces and Moments "/2 -> Bus Element Out1/1
  CG/1 -> "Hydrodynamic Forces and Moments "/4, "Hydrodynamic Forces and Moments "/3
  alpha,beta/1 -> Hydrodynamic Coefficients/1(alpha,beta)
  wb/1 -> Hydrodynamic Coefficients/2(wb)
  Hydrodynamic Coefficients/1(Coeff) -> "Hydrodynamic Forces and Moments "/1
  "Hydrodynamic Forces and Moments "/1 -> Scope/1, Bus Element Out/1

== system AUV_Multi_MPC/Hydrostatic & Hydrodynamic Effects/Underwater Current Forces ==
  note: NOTE:
      | Underwater current velocity is modeled as a first order Markov-like process with a positive
      | time constant m driven by white noise s .
      | Current velocity vector orientation is defined with respect to the World NED reference frame.
  Ground : Ground
  Ground1 : Ground
  Terminator : Terminator
  Terminator1 : Terminator
  Terminator2 : Terminator
  Vcx : Constant  Value=0
  Vcy : Constant  Value=0
  Vcz : Constant  Value=0
  Bus Element Out : Outport  PortName=UnderwaterCurrent  Element=UCForcesXYZ
  Bus Element Out1 : Outport  PortName=UnderwaterCurrent  Element=UCMomentsXYZ
  wires:
  Vcx/1 -> Terminator/1
  Vcy/1 -> Terminator1/1
  Vcz/1 -> Terminator2/1
  Ground/1 -> Bus Element Out/1
  Ground1/1 -> Bus Element Out1/1
